simulink library "rotations_lib"  (R2021a)
settings: Solver=VariableStepAuto  StartTime=0.0  StopTime=10.0  RelTol=1e-3
settings Model: Creator=Nabil  LastModifiedBy=Nabil

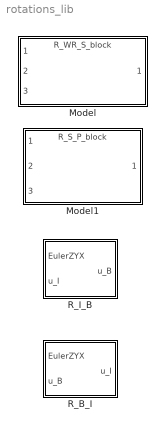
== system rotations_lib ==
  Model : ModelReference  ModelNameDialog=R_WR_S_block.slx  SimulationMode=Normal  ModelReferenceVersion=1.3
  Model1 : ModelReference  ModelNameDialog=R_S_P_block.slx  SimulationMode=Normal  ModelReferenceVersion=1.4
  R_B_I : Subsystem
  R_I_B : Subsystem

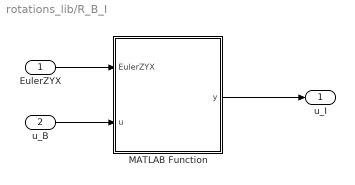
== system rotations_lib/R_B_I ==
  EulerZYX : Inport
  u_B : Inport  Port=2  PortDimensions=3
  MATLAB Function : MATLAB Function  TreatAsAtomicUnit=on
  u_I : Outport
  wires:
  EulerZYX/1 -> MATLAB Function/1(EulerZYX)
  MATLAB Function/1(y) -> u_I/1
  u_B/1 -> MATLAB Function/2(u)

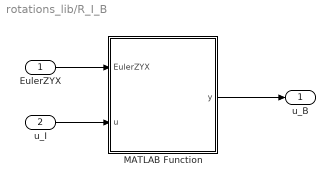
== system rotations_lib/R_I_B ==
  EulerZYX : Inport
  u_I : Inport  Port=2  PortDimensions=3
  MATLAB Function : MATLAB Function  TreatAsAtomicUnit=on
  u_B : Outport
  wires:
  MATLAB Function/1(y) -> u_B/1
  u_I/1 -> MATLAB Function/2(u)
  EulerZYX/1 -> MATLAB Function/1(EulerZYX)

== matlab function rotations_lib/R_I_B/MATLAB Function ==
  data: EulerZYX input; u input; y output
function y = R_I_B(EulerZYX, u)

psi   = EulerZYX(1);
theta = EulerZYX(2);
phi   = EulerZYX(3);

R = rotx(phi)*roty(theta)*rotz(psi);

y = R*u;

end

== matlab function rotations_lib/R_B_I/MATLAB Function ==
  data: EulerZYX input; u input; y output
function y = R_B_I(EulerZYX, u)

psi   = EulerZYX(1);
theta = EulerZYX(2);
phi   = EulerZYX(3);

R = rotx(phi)*roty(theta)*rotz(psi);
y = R/u;

end
